simulink model "ad9361"  (R2015a)
settings: Solver=ode45  StartTime=0.0  StopTime=1  RelTol=1e-3
PreLoadFcn:
  | % newModeS = resample(double(ModeS),25,4);
  | load('newModeS.mat');
  | n = length(newModeS);
libraries: simeventslib x1, dspsrcs4 x1
settings Model: CovSFcnEnable=off  Creator=ACozma  LastModifiedBy=DPu1
settings DebuggingCC: UnderspecifiedInitializationDetection=Classic  MergeDetectMultiDrivingBlocksExec=none  SolverPrmCheckMsg=warning

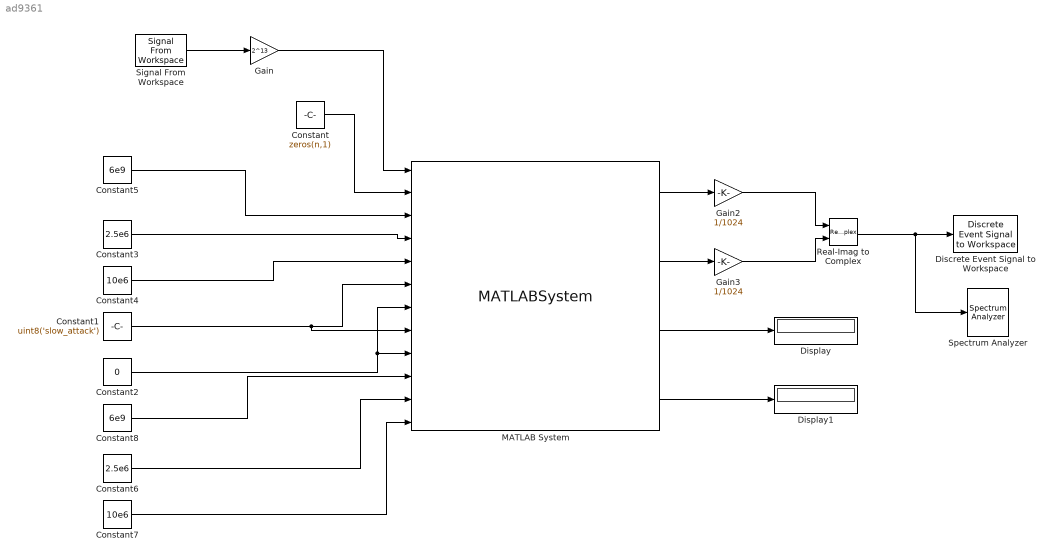
== system ad9361 ==
  Constant : Constant  Value=zeros(n,1)  VectorParams1D=off  FramePeriod=(1e-6/2.5)*n
      settings: SamplingMode=Frame based
  Constant1 : Constant  Value=uint8('slow_attack')  SampleTime=-1
  Constant2 : Constant  Value=0  SampleTime=-1
  Constant3 : Constant  Value=2.5e6  SampleTime=-1
  Constant4 : Constant  Value=10e6  SampleTime=-1
  Constant5 : Constant  Value=6e9  SampleTime=-1
  Constant6 : Constant  Value=2.5e6  SampleTime=-1
  Constant7 : Constant  Value=10e6  SampleTime=-1
  Constant8 : Constant  Value=6e9  SampleTime=-1
  Discrete Event Signal to Workspace : simeventslib/SimEvents Sinks/Discrete Event Signal to Workspace  VariableName=Rx  SaveFormat=Array  isMonitorOnly=off  isRecordIC=off
      settings: MaxDataPoints=n
  Display : Display
  Display1 : Display
  Gain : Gain  Gain=2^13
  Gain2 : Gain  Gain=1/1024
  Gain3 : Gain  Gain=1/1024
  MATLAB System : MATLABSystem  DialogController=sysobjdialog.BlockDynDialog  System=iio_sys_obj  ip_address=192.168.10.2  dev_name=ad9361  in_ch_no=2  in_ch_size=n  out_ch_no=2  out_ch_size=n  SimulateUsing=Interpreted execution
      mask Type: iio_sys_obj
      mask Display:
      | disp('ad9361');
      | port_label('input',1,'DATA_IN1');
      | port_label('input',2,'DATA_IN2');
      | port_label('input',3,'RX_LO_FREQ');
      | port_label('input',4,'RX_SAMPLING_FREQ');
      | port_label('input',5,'RX_RF_BANDWIDTH');
      | port_label('input',6,'RX1_GAIN_MODE');
      | port_label('input',7,'RX1_GAIN');
      | port_label('input',8,'RX2_GAIN_MODE');
      | port_label('input',9,'RX2_GAIN');
      | port_label('input',10,'TX_LO_FREQ');
      | port_label('input',11,'TX_SAMPLING_FREQ');
      | port_label('input',12,'TX_RF_BANDWIDTH');
      | port_label('output',1,'DATA_OUT1');
      | port_label('output',2,'DATA_OUT2');
      | port_label('output',3,'RX1_RSSI');
      | port_label('output',4,'RX2_RSSI');
  Real-Imag to Complex : RealImagToComplex
  Signal From Workspace : dspsrcs4/Signal From Workspace  X=newModeS  Ts=1e-6/(2.5)  nsamps=n  OutputAfterFinalValue=Cyclic repetition  ignoreOrWarnInputAndFrameLengths=off
  Spectrum Analyzer : SpectrumAnalyzer
  wires:
  MATLAB System/3 -> Display/1
  MATLAB System/4 -> Display1/1
  Constant5/1 -> MATLAB System/3
  Constant3/1 -> MATLAB System/4
  Constant4/1 -> MATLAB System/5
  Constant1/1 -> MATLAB System/8, MATLAB System/6
  Constant2/1 -> MATLAB System/9, MATLAB System/7
  Constant8/1 -> MATLAB System/10
  Constant6/1 -> MATLAB System/11
  Constant7/1 -> MATLAB System/12
  Gain2/1 -> Real-Imag to Complex/1
  MATLAB System/1 -> Gain2/1
  MATLAB System/2 -> Gain3/1
  Gain/1 -> MATLAB System/1
  Signal From Workspace/1 -> Gain/1
  Constant/1 -> MATLAB System/2
  Gain3/1 -> Real-Imag to Complex/2
  Real-Imag to Complex/1 -> Spectrum Analyzer/1, Discrete Event Signal to Workspace/1
